simulink model "classActivity (2)"  (R2023b)
settings: Solver=FixedStepAuto  StartTime=0.0  StopTime=10.0  FixedStep=0.01  RelTol=1e-3
libraries: arduinolib x7, simulink x3
settings Model: ExtModeTrigDuration=2  Creator=qasem  LastModifiedBy=qasem
settings OptimizationCC: EnhancedBackFolding=on  PassReuseOutputArgsAs=Individual arguments  ZeroExternalMemoryAtStartup=off  ZeroInternalMemoryAtStartup=off  MaxStackSize=64  OptimizeBlockOrder=speed  DifferentSizesBufferReuse=on  OptimizationCustomize=off  EfficientTunableParamExpr=on
settings DebuggingCC: ParameterTunabilityLossMsg=error
settings HardwareCC: ProdBitPerInt=16  ProdBitPerPointer=16  ProdBitPerSizeT=16  ProdBitPerPtrDiffT=16  ProdLargestAtomicFloat=None  ProdWordSize=8  ProdHWDeviceType=Atmel->AVR
settings SFSimCC: MATLABDynamicMemAlloc=off
settings RTWCC: Description=Embedded Coder  SystemTargetFile=ert.tlc  HardwareBoard=Arduino Mega 2560  TemplateMakefile=ert_default_tmf  Toolchain=Arduino AVR
settings CodeAppCC: ForceParamTrailComments=on  IgnoreCustomStorageClasses=off  OperatorAnnotations=on  SimulinkDataObjDesc=on  SFDataObjDesc=on  InsertBlockDesc=on
settings ERTTargetCC: SupportContinuousTime=on  SupportVariableSizeSignals=on  ExtModeTransport=3  ExtModeStaticAlloc=on  ExtModeAutomaticAllocSize=off  ExtModeStaticAllocSize=2048  ExtModeMexFile=ext_xcp  ExtModeIntrfLevel=Level2 - Open

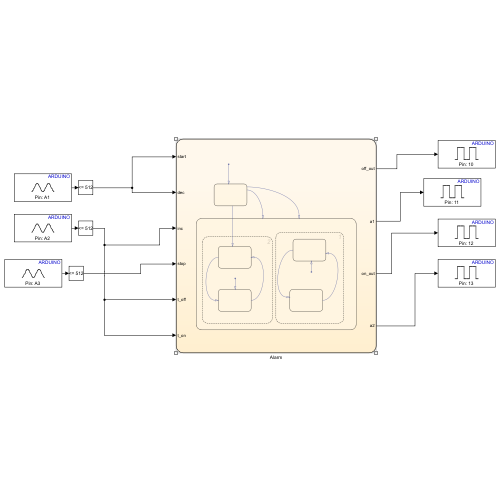
[thumbnail: Simulink's stored preview of the top-level diagram]
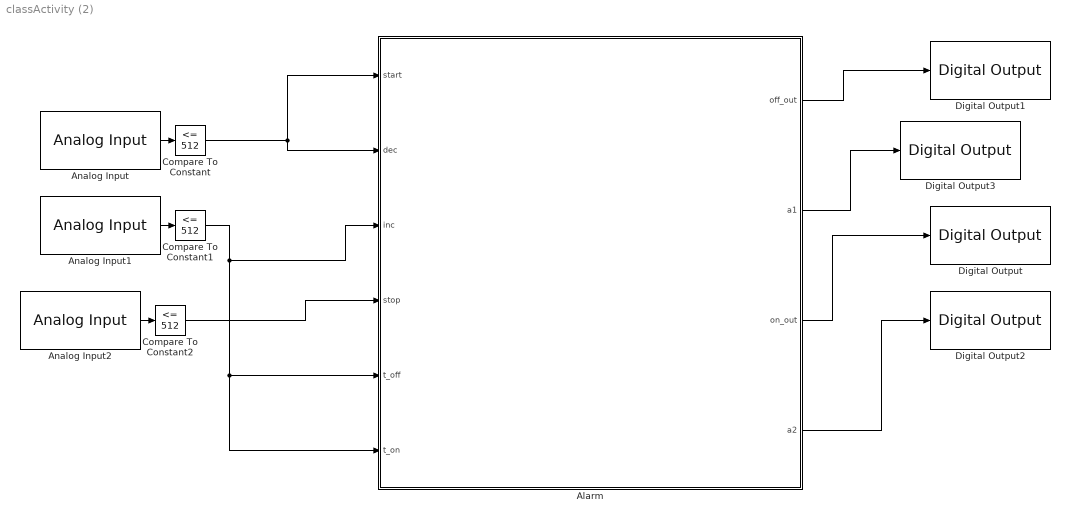
== system classActivity (2) ==
  Alarm : Stateflow chart  TreatAsAtomicUnit=on
      settings: PortSchema="{\"entries\":[{\"content\":{\"sides\":[{\"content\":{\"connectorIds\":[\"In1\",\"In2\",\"In3\",\"In4\",\"In5\",\"In6\"]},\"type\":\"ConnectorPlacement.EquallySpacedRectSide\",\"uuid\":\"67fa7592-dd5f-473b-adb5-31a8a36dc656\"},{\"content\":{\"connectorIds\":[\"Out1\",\"Out3\",\"Out2\",\"Out4\"],\"side\":\"RIGHT\"},\"type\":\"ConnectorPlacement.EquallySpacedRectSide\",\"uuid\":\"ab42aef1-4252-4a8b-8856-fd08774fb9b6\"},{\"content\":{\"side\":\"TOP\"},\"type\":\"ConnectorPlacement.EquallySpacedRectSide\",\"uuid\":\"0f3ec35b-95fb-46bd-8956-4d67cc055612\"}]},\"type\":\"ConnectorPlacement.EquallySpacedConnector\",\"uuid\":\"eed7d48e-0090-434b-a77a-4ae4108e4a5f\"}],\"packageUris\":[\"http://schema.mathworks.com/mf0/Connector/R2020b\"],\"version\":\"1.0\"}"
  Analog Input : arduinolib/Analog Input  pinNumber=1  ReadResultsOnly=off  ConversionTriggerSource=Software  ExternalTriggerType=uint32( 0 )  OutputDataType=uint16  EnableConversionCompleteNotify=off  EnableOuputStatus=off  SampleTime=-1  blockPlatform=arduino
  Analog Input1 : arduinolib/Analog Input  pinNumber=2  ReadResultsOnly=off  ConversionTriggerSource=Software  ExternalTriggerType=uint32( 0 )  OutputDataType=uint16  EnableConversionCompleteNotify=off  EnableOuputStatus=off  SampleTime=-1  blockPlatform=arduino
  Analog Input2 : arduinolib/Analog Input  pinNumber=3  ReadResultsOnly=off  ConversionTriggerSource=Software  ExternalTriggerType=uint32( 0 )  OutputDataType=uint16  EnableConversionCompleteNotify=off  EnableOuputStatus=off  SampleTime=-1  blockPlatform=arduino
  Compare To Constant : simulink/Logic and Bit Operations/Compare To Constant  relop=<=  const=512  OutDataTypeStr=boolean
  Compare To Constant1 : simulink/Logic and Bit Operations/Compare To Constant  relop=<=  const=512  OutDataTypeStr=boolean
  Compare To Constant2 : simulink/Logic and Bit Operations/Compare To Constant  relop=<=  const=512  OutDataTypeStr=boolean
  Digital Output : arduinolib/Digital Output  pinNumber=12  Direction=output  blockPlatform=arduino
  Digital Output1 : arduinolib/Digital Output  pinNumber=10  Direction=output  blockPlatform=arduino
  Digital Output2 : arduinolib/Digital Output  pinNumber=13  Direction=output  blockPlatform=arduino
  Digital Output3 : arduinolib/Digital Output  pinNumber=11  Direction=output  blockPlatform=arduino
  wires:
  Compare To Constant/1 -> Alarm/2(dec), Alarm/1(start)
  Compare To Constant1/1 -> Alarm/3(inc), Alarm/5(t_off), Alarm/6(t_on)
  Alarm/2(on_out) -> Digital Output/1
  Alarm/3(a1) -> Digital Output3/1
  Alarm/4(a2) -> Digital Output2/1
  Analog Input/1 -> Compare To Constant/1
  Analog Input1/1 -> Compare To Constant1/1
  Alarm/1(off_out) -> Digital Output1/1
  Analog Input2/1 -> Compare To Constant2/1
  Compare To Constant2/1 -> Alarm/4(stop)

== stateflow chart classActivity (2)/Alarm ==
  state Shutdown
  state OP
    state Vol [parallel]
      settings: executionOrder=1
      state One
        entry:a1 = true;
        exit: a1 = false;
      state Two
        entry: a2 = true;
        exit: a2 = false;
      One -> Two : [inc==true]
      Two -> One : [dec==true]
      (default) -> One
    state Mode [parallel]
      settings: executionOrder=2
      state ON
        entry:
        on_out = true;
        exit: on_out =false;
      state Off
        entry:
        off_out = true;
        exit: off_out = false;
      Off -> ON : [t_on==true]
      ON -> Off : [t_off==true]
      (default) -> Off
  (default) -> Shutdown
  Shutdown -> OP [order 1] : [stop ==true]
  Shutdown -> OP [order 2] : [start == true]
  Shutdown -> ON [order 3] : [t_on==true]
  data: start input boolean; dec input boolean; inc input boolean; stop input boolean; t_off input boolean; t_on input boolean; off_out output boolean; on_out output boolean; a1 output boolean; a2 output boolean
